simulink model "test_optimization"  (R2014b)
settings: Solver=VariableStepDiscrete  StartTime=0.0  StopTime=100  RelTol=1e-3
undefined symbols (not defined in the file): h, sys_d
libraries: simulink x1
settings Model: Creator=mlab-retro  LastModifiedBy=mlab-retro

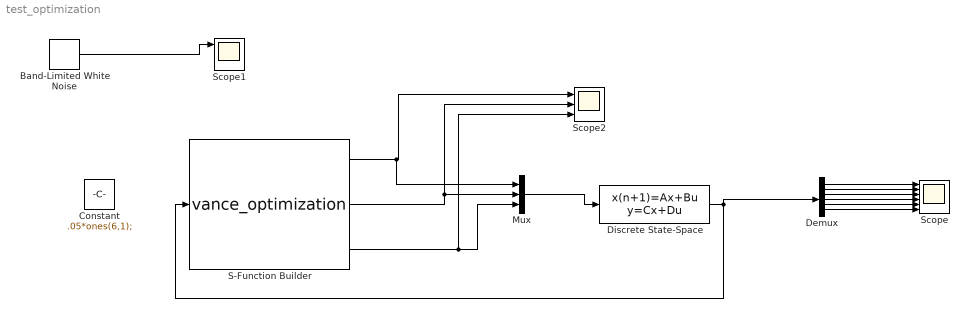
== system test_optimization ==
  Band-Limited White Noise : simulink/Sources/Band-Limited White Noise  Cov=[0.01,0.02,0.01,0.01,0.01,0.005]  Ts=0.1  seed=[23341,13243,11231,27867,34551,12317]
  Constant : Constant  Value=.05*ones(6,1);
  Demux : Demux  Outputs=6
  Discrete State-Space : DiscreteStateSpace  A=sys_d.a  B=sys_d.b  C=sys_d.c  D=sys_d.d  X0=[10;10;10;0;0;0];  SampleTime=h
  Mux : Mux  Inputs=3
  S-Function Builder : S-Function  InitFcn=try, set_param(gcb,'FunctionName','vance_optimization'), end  FunctionName=vance_optimization  SFunctionModules=vance_optimization_wrapper ldl matrix_support solver util  EnableBusSupport=off  mask(S-Function Builder){}
      mask help: Simulink:masks:SFunctionBuilder_MD
      mask init:
      | val = [[.9  0.75 0.75 1 1 .9 .9 1]',[1 1 0.75 0.75 .9 .9 1 .9]'];try , sys = get_param(gcb,'SfunBuilderFcnName');if isempty(sys), sys = get_param(gcb,'FunctionName'); end,catch, sys = get_param(gcb,'FunctionName'); end
      settings: CopyFcn=set_param(gcbh,'LinkStatus','none')  PreSaveFcn=try, set_param(gcb,'FunctionName','vance_optimization'), end  OpenFcn=sfunctionwizard(gcbh)
      mask Display:
      | plot(val(:,1),val(:,2))
      | disp(sys)
      | port_label('input',1,'x_hat')
      | port_label('output',1,'theta')
      | port_label('output',2,'phi')
      | port_label('output',3,'thrust')
  Scope : Scope  NumInputPorts=6
      settings: YMin=-5~-5~-5~-5~-5~-5  YMax=5~5~5~5~5~5
  Scope1 : Scope  NumInputPorts=3
      settings: YMin=-5~-5~-5  YMax=5~5~5
  Scope2 : Scope  NumInputPorts=3
      settings: YMin=-5~-5~-5  YMax=5~5~5  SaveName=ScopeData2
  wires:
  Band-Limited White Noise/1 -> Scope1/1
  S-Function Builder/1 -> Mux/1, Scope2/1
  Mux/1 -> Discrete State-Space/1
  S-Function Builder/2 -> Mux/2, Scope2/2
  S-Function Builder/3 -> Scope2/3, Mux/3
  Discrete State-Space/1 -> S-Function Builder/1, Demux/1
  Demux/2 -> Scope/2
  Demux/4 -> Scope/4
  Demux/1 -> Scope/1
  Demux/3 -> Scope/3
  Demux/5 -> Scope/5
  Demux/6 -> Scope/6
